simulink model "PM_fnc11_TestHarness2"  (R2022a)
settings: Solver=FixedStepDiscrete  StartTime=1  StopTime=inf  FixedStep=1  RelTol=1e-3
values from neighbouring files (symbols this model uses):
  fixedsteprate_s = rate_s    (= 0.01)    [PM_fnc1000_tc01_iter01_testsignal_builder.m]    (also in PM_fnc21_tc01_iter01_testsignal_builder.m; PM_fnc22_tc01_iter01_testsignal_builder.m)
undefined symbols (not defined in the file or in its folder): cal_DchgPL1_expiry_dur_thresh_ms, cal_DchgPL1_restore_dur_thresh_ms
settings Model: PacingRate=1.500000  Creator=306427  LastModifiedBy=306427
settings SolverCC: ZeroCrossAlgorithm=Adaptive

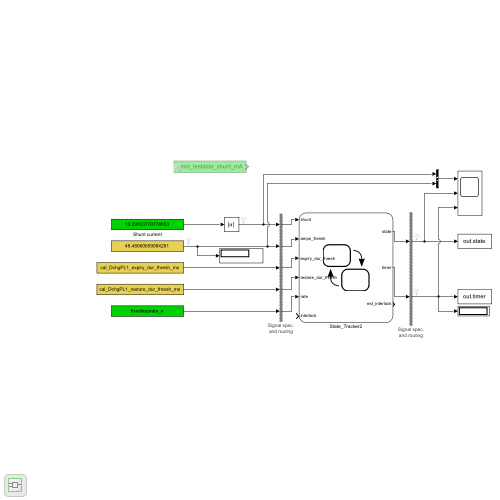
[thumbnail: Simulink's stored preview of the top-level diagram]
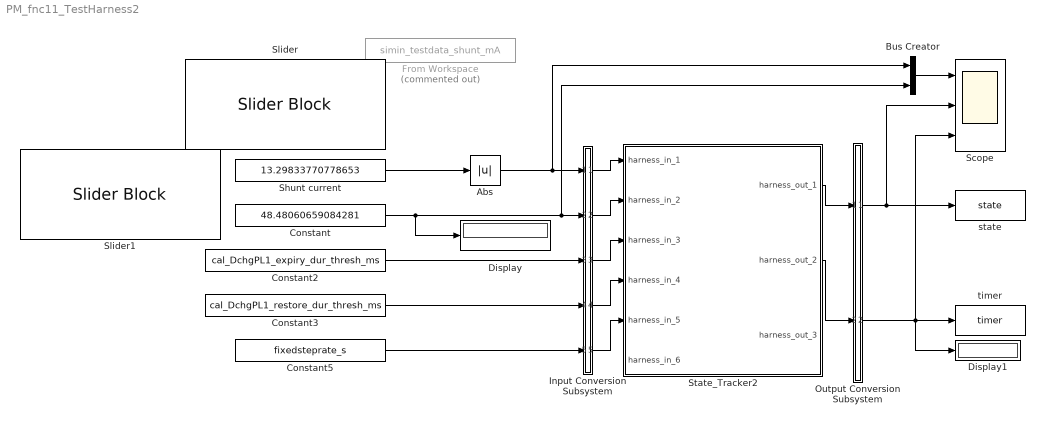
== system PM_fnc11_TestHarness2 ==
  Abs : Abs  SaturateOnIntegerOverflow=off
  Bus Creator : BusCreator  Inputs=2
  Constant : Constant  Value=48.48060659084281
  Constant2 : Constant  Value=cal_DchgPL1_expiry_dur_thresh_ms
  Constant3 : Constant  Value=cal_DchgPL1_restore_dur_thresh_ms
  Constant5 : Constant  Value=fixedsteprate_s
  Display : Display
  Display1 : Display
  From Workspace : FromWorkspace  Commented=on  VariableName=simin_testdata_shunt_mA
  Input Conversion Subsystem : Subsystem  Tag=__SLT_ICS__  Description=|
      | Signal spec.
      | and routing
      settings: AttributesFormatString=%<Description>
  Output Conversion Subsystem : Subsystem  Tag=__SLT_OCS__  Description=|
      | Signal spec.
      | and routing
      settings: AttributesFormatString=%<Description>
  Scope : Scope  NumInputPorts=3
  Shunt current : Constant  Value=13.29833770778653
  Slider : SliderBlock  ScaleMax=300
  Slider1 : SliderBlock
  State_Tracker2 : Subsystem  Tag=__SL_testing_harness_stub_
  state : ToWorkspace  VariableName=state  SaveFormat=Timeseries
  timer : ToWorkspace  VariableName=timer  SaveFormat=Timeseries
  wires:
  Shunt current/1 -> Abs/1
  Output Conversion Subsystem/1(Outport_1) -> Scope/2, state/1
  Output Conversion Subsystem/2(Outport_2) -> Display1/1, Scope/3, timer/1
  Input Conversion Subsystem/1(Outport_1) -> State_Tracker2/1(harness_in_1)
  Input Conversion Subsystem/2(Outport_2) -> State_Tracker2/2(harness_in_2)
  Input Conversion Subsystem/3(Outport_3) -> State_Tracker2/3(harness_in_3)
  Input Conversion Subsystem/4(Outport_4) -> State_Tracker2/4(harness_in_4)
  Input Conversion Subsystem/5(Outport_5) -> State_Tracker2/5(harness_in_5)
  State_Tracker2/1(harness_out_1) -> Output Conversion Subsystem/1(Inport_1)
  State_Tracker2/2(harness_out_2) -> Output Conversion Subsystem/2(Inport_2)
  Constant/1 -> Display/1, Bus Creator/2, Input Conversion Subsystem/2(Inport_2)
  Constant2/1 -> Input Conversion Subsystem/3(Inport_3)
  Constant3/1 -> Input Conversion Subsystem/4(Inport_4)
  Constant5/1 -> Input Conversion Subsystem/5(Inport_5)
  Abs/1 -> Input Conversion Subsystem/1(Inport_1), Bus Creator/1
  Bus Creator/1 -> Scope/1

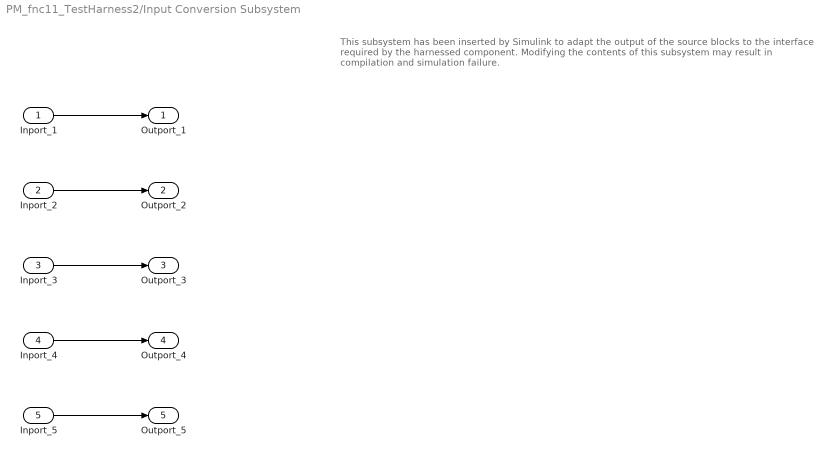
== system PM_fnc11_TestHarness2/Input Conversion Subsystem ==
  note: This subsystem has been inserted by Simulink to adapt the output of the source blocks to the interface required by the harnessed component.
      |  Modifying the contents of this subsystem may result in compilation and simulation failure.
  Inport_1 : Inport
  Inport_2 : Inport  Port=2
  Inport_3 : Inport  Port=3
  Inport_4 : Inport  Port=4
  Inport_5 : Inport  Port=5
  Outport_1 : Outport
  Outport_2 : Outport  Port=2
  Outport_3 : Outport  Port=3
  Outport_4 : Outport  Port=4
  Outport_5 : Outport  Port=5
  wires:
  Inport_1/1 -> Outport_1/1
  Inport_2/1 -> Outport_2/1
  Inport_3/1 -> Outport_3/1
  Inport_4/1 -> Outport_4/1
  Inport_5/1 -> Outport_5/1

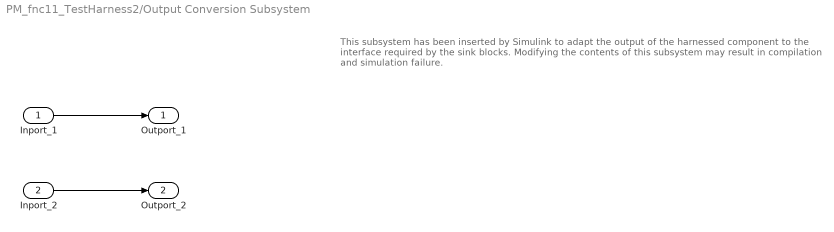
== system PM_fnc11_TestHarness2/Output Conversion Subsystem ==
  note: This subsystem has been inserted by Simulink to adapt the output of the harnessed component to the interface required by the sink blocks.
      |  Modifying the contents of this subsystem may result in compilation and simulation failure.
  Inport_1 : Inport
  Inport_2 : Inport  Port=2
  Outport_1 : Outport
  Outport_2 : Outport  Port=2
  wires:
  Inport_1/1 -> Outport_1/1
  Inport_2/1 -> Outport_2/1

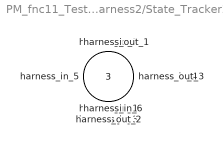
== system PM_fnc11_TestHarness2/State_Tracker2 ==
  harness_in_1 : Inport
  harness_in_2 : Inport  Port=2
  harness_in_3 : Inport  Port=3
  harness_in_4 : Inport  Port=4
  harness_in_5 : Inport  Port=5
  harness_in_6 : Inport  Port=6
  harness_out_1 : Outport
  harness_out_2 : Outport  Port=2
  harness_out_3 : Outport  Port=3
